simulink model "LgrstClsRStEnCtrl"  (R2018b)
settings: Solver=FixedStepDiscrete  StartTime=0.0  StopTime=10.0  FixedStep=0.01  RelTol=1e-3
undefined symbols (not defined in the file or in its folder): data, KeSMSw4SSecRwRtStLgrstOtwdInwdClosePos1_Val, KeSMSw4SSecRwRtStLgrstUpwdDnwdClosePos1_Val, KeSMSw4SSecRwRtStLgrstUpwdDnwdClosePos2_Val, SecRwRtStFtrstEn_Clear, SecRwRtStFtrstEn_Set, SecRwRtStLgrstInwdOtwdEn_Clear, SecRwRtStLgrstInwdOtwdEn_Set, SecRwRtStLgrstUpwdDnwdEn_Clear, SecRwRtStLgrstUpwdDnwdEn_Set
libraries: simulink x7
settings Model: Creator=sn2xws  LastModifiedBy=sn2xws
settings DataIOCC: SaveFormat=StructureWithTime
settings OptimizationCC: DefaultParameterBehavior=Inlined  EnhancedBackFolding=on  PassReuseOutputArgsAs=Individual arguments  ZeroExternalMemoryAtStartup=off  ZeroInternalMemoryAtStartup=off  OptimizeBlockOrder=speed  DifferentSizesBufferReuse=on  OptimizationCustomize=off
settings DebuggingCC: ParameterTunabilityLossMsg=error
settings ModelReferenceCC: ModelReferenceNumInstancesAllowed=Single
settings SFSimCC: MATLABDynamicMemAlloc=off
settings RTWCC: SystemTargetFile=autosar.tlc  GenCodeOnly=on  TemplateMakefile=ert_default_tmf  Description=AUTOSAR  GenerateReport=on  IncludeHyperlinkInReport=on  LaunchReport=on  GenerateTraceInfo=on  GenerateTraceReport=on  GenerateTraceReportSl=on  GenerateTraceReportSf=on  GenerateTraceReportEml=on
settings CodeAppCC: ForceParamTrailComments=on  IgnoreCustomStorageClasses=off  OperatorAnnotations=on  SimulinkDataObjDesc=on  SFDataObjDesc=on  InsertBlockDesc=on
settings STFCustomTargetCC: TargetLangStandard=C99 (ISO)  MultiwordLength=256  ParMdlRefBuildCompliant=on  CompOptLevelCompliant=on  IncludeMdlTerminateFcn=off  CombineOutputUpdateFcns=on  SuppressErrorStatus=on  ERTCustomFileBanners=on  SupportNonFinite=off  SupportComplex=off  SupportContinuousTime=off  SupportNonInlinedSFcns=off  RemoveResetFunc=on  MATLABClassNameForMDSCustomization=Simulink.SoftwareTarget.ERTCustomization  AutosarCompliant=on  UseToolchainInfoCompliant=on  LookupTableObjectStructAxisOrder=2,1,3,4,...  LUTObjectStructOrderEvenSpacing=Size,Table,Breakpoints  SystemTargetFile=autosar.tlc
settings ERTTargetCC: TargetLangStandard=C99 (ISO)  ConcurrentExecutionCompliant=off  IncludeMdlTerminateFcn=off  SuppressErrorStatus=on  SupportNonFinite=off  SupportComplex=off  ModelStepFunctionPrototypeControlCompliant=off  CPPClassGenCompliant=off  AutosarCompliant=on  LookupTableObjectStructAxisOrder=2,1,3,4,...  LUTObjectStructOrderEvenSpacing=Size,Table,Breakpoints  InlinedParameterPlacement=NonHierarchical  ERTCustomFileTemplate=example_file_process.tlc  ERTFilePackagingFormat=Compact

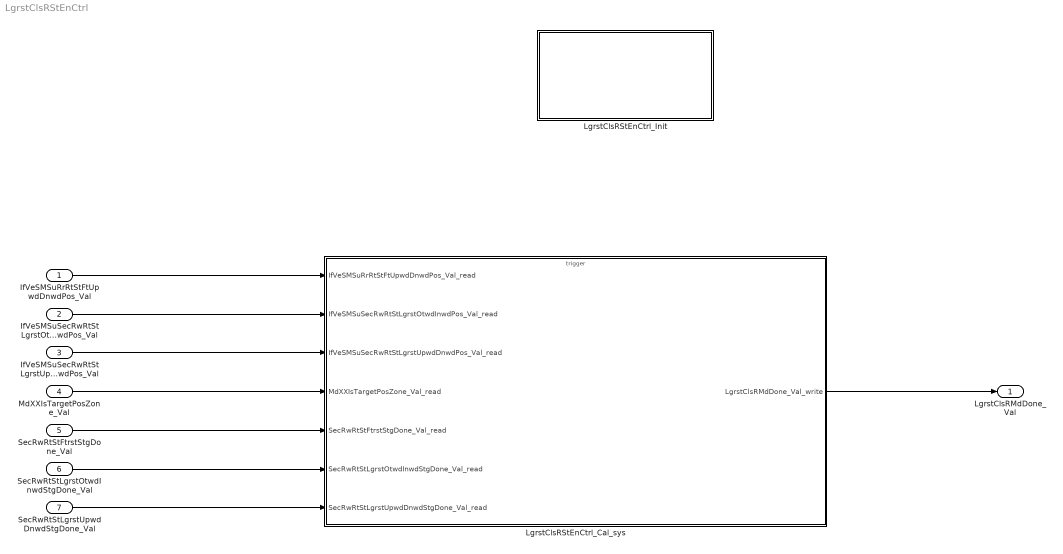
== system LgrstClsRStEnCtrl ==
  IfVeSMSuRrRtStFtUpwdDnwdPos_Val : Inport  OutDataTypeStr=uint16  PortDimensions=1
  IfVeSMSuSecRwRtStLgrstOtwdInwdPos_Val : Inport  Port=2  OutDataTypeStr=uint16  PortDimensions=1
  IfVeSMSuSecRwRtStLgrstUpwdDnwdPos_Val : Inport  Port=3  OutDataTypeStr=uint16  PortDimensions=1
  MdXXIsTargetPosZone_Val : Inport  Port=4  OutDataTypeStr=uint32  PortDimensions=1
  SecRwRtStFtrstStgDone_Val : Inport  Port=5  OutDataTypeStr=boolean  PortDimensions=1
  SecRwRtStLgrstOtwdInwdStgDone_Val : Inport  Port=6  OutDataTypeStr=boolean  PortDimensions=1
  SecRwRtStLgrstUpwdDnwdStgDone_Val : Inport  Port=7  OutDataTypeStr=boolean  PortDimensions=1
  LgrstClsRStEnCtrl_Cal_sys : Subsystem
  LgrstClsRStEnCtrl_Init : Subsystem
  LgrstClsRMdDone_Val : Outport  OutDataTypeStr=uint8  PortDimensions=1
  wires:
  IfVeSMSuRrRtStFtUpwdDnwdPos_Val/1 -> LgrstClsRStEnCtrl_Cal_sys/1(IfVeSMSuRrRtStFtUpwdDnwdPos_Val_read)
  IfVeSMSuSecRwRtStLgrstOtwdInwdPos_Val/1 -> LgrstClsRStEnCtrl_Cal_sys/2(IfVeSMSuSecRwRtStLgrstOtwdInwdPos_Val_read)
  IfVeSMSuSecRwRtStLgrstUpwdDnwdPos_Val/1 -> LgrstClsRStEnCtrl_Cal_sys/3(IfVeSMSuSecRwRtStLgrstUpwdDnwdPos_Val_read)
  MdXXIsTargetPosZone_Val/1 -> LgrstClsRStEnCtrl_Cal_sys/4(MdXXIsTargetPosZone_Val_read)
  SecRwRtStFtrstStgDone_Val/1 -> LgrstClsRStEnCtrl_Cal_sys/5(SecRwRtStFtrstStgDone_Val_read)
  SecRwRtStLgrstOtwdInwdStgDone_Val/1 -> LgrstClsRStEnCtrl_Cal_sys/6(SecRwRtStLgrstOtwdInwdStgDone_Val_read)
  SecRwRtStLgrstUpwdDnwdStgDone_Val/1 -> LgrstClsRStEnCtrl_Cal_sys/7(SecRwRtStLgrstUpwdDnwdStgDone_Val_read)
  LgrstClsRStEnCtrl_Cal_sys/1(LgrstClsRMdDone_Val_write) -> LgrstClsRMdDone_Val/1

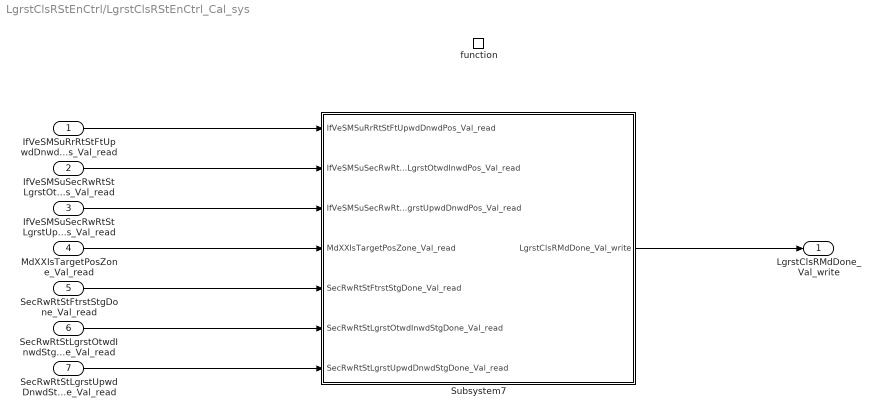
== system LgrstClsRStEnCtrl/LgrstClsRStEnCtrl_Cal_sys ==
  IfVeSMSuRrRtStFtUpwdDnwdPos_Val_read : Inport
  IfVeSMSuSecRwRtStLgrstOtwdInwdPos_Val_read : Inport  Port=2
  IfVeSMSuSecRwRtStLgrstUpwdDnwdPos_Val_read : Inport  Port=3
  MdXXIsTargetPosZone_Val_read : Inport  Port=4
  SecRwRtStFtrstStgDone_Val_read : Inport  Port=5
  SecRwRtStLgrstOtwdInwdStgDone_Val_read : Inport  Port=6
  SecRwRtStLgrstUpwdDnwdStgDone_Val_read : Inport  Port=7
  function : TriggerPort  TriggerType=function-call  IsSimulinkFunction=on  FunctionName=LgrstClsRStEnCtrl_Cal  VariantControl=(inherit)
  Subsystem7 : Subsystem
  LgrstClsRMdDone_Val_write : Outport
      settings: EnsureOutportIsVirtual=on
  wires:
  IfVeSMSuRrRtStFtUpwdDnwdPos_Val_read/1 -> Subsystem7/1(IfVeSMSuRrRtStFtUpwdDnwdPos_Val_read)
  IfVeSMSuSecRwRtStLgrstOtwdInwdPos_Val_read/1 -> Subsystem7/2(IfVeSMSuSecRwRtStLgrstOtwdInwdPos_Val_read)
  IfVeSMSuSecRwRtStLgrstUpwdDnwdPos_Val_read/1 -> Subsystem7/3(IfVeSMSuSecRwRtStLgrstUpwdDnwdPos_Val_read)
  MdXXIsTargetPosZone_Val_read/1 -> Subsystem7/4(MdXXIsTargetPosZone_Val_read)
  SecRwRtStFtrstStgDone_Val_read/1 -> Subsystem7/5(SecRwRtStFtrstStgDone_Val_read)
  SecRwRtStLgrstOtwdInwdStgDone_Val_read/1 -> Subsystem7/6(SecRwRtStLgrstOtwdInwdStgDone_Val_read)
  SecRwRtStLgrstUpwdDnwdStgDone_Val_read/1 -> Subsystem7/7(SecRwRtStLgrstUpwdDnwdStgDone_Val_read)
  Subsystem7/1(LgrstClsRMdDone_Val_write) -> LgrstClsRMdDone_Val_write/1

== system LgrstClsRStEnCtrl/LgrstClsRStEnCtrl_Init ==
  Event Listener : EventListener  EventName=reset

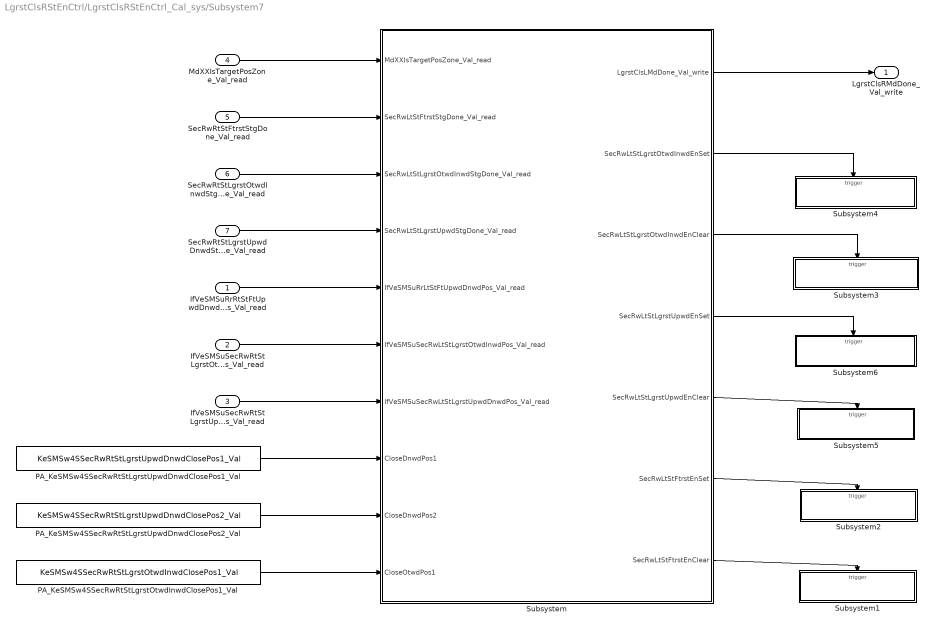
== system LgrstClsRStEnCtrl/LgrstClsRStEnCtrl_Cal_sys/Subsystem7 ==
  IfVeSMSuRrRtStFtUpwdDnwdPos_Val_read : Inport
  IfVeSMSuSecRwRtStLgrstOtwdInwdPos_Val_read : Inport  Port=2
  IfVeSMSuSecRwRtStLgrstUpwdDnwdPos_Val_read : Inport  Port=3
  MdXXIsTargetPosZone_Val_read : Inport  Port=4
  SecRwRtStFtrstStgDone_Val_read : Inport  Port=5
  SecRwRtStLgrstOtwdInwdStgDone_Val_read : Inport  Port=6
  SecRwRtStLgrstUpwdDnwdStgDone_Val_read : Inport  Port=7
  PA_KeSMSw4SSecRwRtStLgrstOtwdInwdClosePos1_Val : Constant  Value=KeSMSw4SSecRwRtStLgrstOtwdInwdClosePos1_Val
  PA_KeSMSw4SSecRwRtStLgrstUpwdDnwdClosePos1_Val : Constant  Value=KeSMSw4SSecRwRtStLgrstUpwdDnwdClosePos1_Val
  PA_KeSMSw4SSecRwRtStLgrstUpwdDnwdClosePos2_Val : Constant  Value=KeSMSw4SSecRwRtStLgrstUpwdDnwdClosePos2_Val
  Subsystem : Subsystem
  Subsystem1 : Subsystem
  Subsystem2 : Subsystem
  Subsystem3 : Subsystem
  Subsystem4 : Subsystem
  Subsystem5 : Subsystem
  Subsystem6 : Subsystem
  LgrstClsRMdDone_Val_write : Outport
      settings: EnsureOutportIsVirtual=on
  wires:
  SecRwRtStLgrstUpwdDnwdStgDone_Val_read/1 -> Subsystem/4(SecRwLtStLgrstUpwdStgDone_Val_read)
  SecRwRtStLgrstOtwdInwdStgDone_Val_read/1 -> Subsystem/3(SecRwLtStLgrstOtwdInwdStgDone_Val_read)
  IfVeSMSuSecRwRtStLgrstUpwdDnwdPos_Val_read/1 -> Subsystem/7(IfVeSMSuSecRwLtStLgrstUpwdDnwdPos_Val_read)
  MdXXIsTargetPosZone_Val_read/1 -> Subsystem/1(MdXXIsTargetPosZone_Val_read)
  Subsystem/1(LgrstClsLMdDone_Val_write) -> LgrstClsRMdDone_Val_write/1
  Subsystem/7(SecRwLtStFtrstEnClear) -> Subsystem1/Trigger
  SecRwRtStFtrstStgDone_Val_read/1 -> Subsystem/2(SecRwLtStFtrstStgDone_Val_read)
  Subsystem/4(SecRwLtStLgrstUpwdEnSet) -> Subsystem6/Trigger
  PA_KeSMSw4SSecRwRtStLgrstUpwdDnwdClosePos2_Val/1 -> Subsystem/9(CloseDnwdPos2)
  Subsystem/2(SecRwLtStLgrstOtwdInwdEnSet) -> Subsystem4/Trigger
  Subsystem/6(SecRwLtStFtrstEnSet) -> Subsystem2/Trigger
  IfVeSMSuRrRtStFtUpwdDnwdPos_Val_read/1 -> Subsystem/5(IfVeSMSuRrLtStFtUpwdDnwdPos_Val_read)
  Subsystem/3(SecRwLtStLgrstOtwdInwdEnClear) -> Subsystem3/Trigger
  IfVeSMSuSecRwRtStLgrstOtwdInwdPos_Val_read/1 -> Subsystem/6(IfVeSMSuSecRwLtStLgrstOtwdInwdPos_Val_read)
  PA_KeSMSw4SSecRwRtStLgrstOtwdInwdClosePos1_Val/1 -> Subsystem/10(CloseOtwdPos1)
  PA_KeSMSw4SSecRwRtStLgrstUpwdDnwdClosePos1_Val/1 -> Subsystem/8(CloseDnwdPos1)
  Subsystem/5(SecRwLtStLgrstUpwdEnClear) -> Subsystem5/Trigger

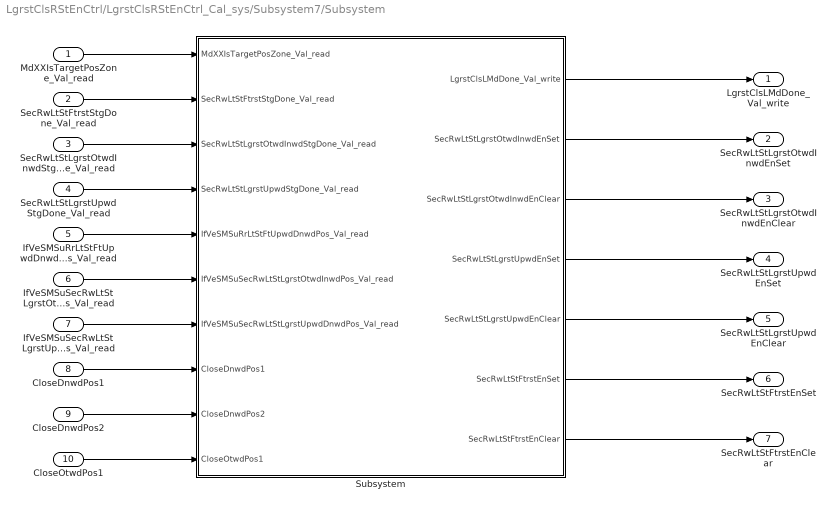
== system LgrstClsRStEnCtrl/LgrstClsRStEnCtrl_Cal_sys/Subsystem7/Subsystem ==
  MdXXIsTargetPosZone_Val_read : Inport
  SecRwLtStFtrstStgDone_Val_read : Inport  Port=2
  SecRwLtStLgrstOtwdInwdStgDone_Val_read : Inport  Port=3
  SecRwLtStLgrstUpwdStgDone_Val_read : Inport  Port=4
  IfVeSMSuRrLtStFtUpwdDnwdPos_Val_read : Inport  Port=5
  IfVeSMSuSecRwLtStLgrstOtwdInwdPos_Val_read : Inport  Port=6
  IfVeSMSuSecRwLtStLgrstUpwdDnwdPos_Val_read : Inport  Port=7
  CloseDnwdPos1 : Inport  Port=8
  CloseDnwdPos2 : Inport  Port=9
  CloseOtwdPos1 : Inport  Port=10
  Subsystem : Subsystem
  LgrstClsLMdDone_Val_write : Outport
      settings: EnsureOutportIsVirtual=on
  SecRwLtStLgrstOtwdInwdEnSet : Outport  Port=2
  SecRwLtStLgrstOtwdInwdEnClear : Outport  Port=3
  SecRwLtStLgrstUpwdEnSet : Outport  Port=4
  SecRwLtStLgrstUpwdEnClear : Outport  Port=5
  SecRwLtStFtrstEnSet : Outport  Port=6
  SecRwLtStFtrstEnClear : Outport  Port=7
  wires:
  MdXXIsTargetPosZone_Val_read/1 -> Subsystem/1(MdXXIsTargetPosZone_Val_read)
  SecRwLtStFtrstStgDone_Val_read/1 -> Subsystem/2(SecRwLtStFtrstStgDone_Val_read)
  SecRwLtStLgrstOtwdInwdStgDone_Val_read/1 -> Subsystem/3(SecRwLtStLgrstOtwdInwdStgDone_Val_read)
  SecRwLtStLgrstUpwdStgDone_Val_read/1 -> Subsystem/4(SecRwLtStLgrstUpwdStgDone_Val_read)
  Subsystem/1(LgrstClsLMdDone_Val_write) -> LgrstClsLMdDone_Val_write/1
  IfVeSMSuSecRwLtStLgrstOtwdInwdPos_Val_read/1 -> Subsystem/6(IfVeSMSuSecRwLtStLgrstOtwdInwdPos_Val_read)
  IfVeSMSuRrLtStFtUpwdDnwdPos_Val_read/1 -> Subsystem/5(IfVeSMSuRrLtStFtUpwdDnwdPos_Val_read)
  IfVeSMSuSecRwLtStLgrstUpwdDnwdPos_Val_read/1 -> Subsystem/7(IfVeSMSuSecRwLtStLgrstUpwdDnwdPos_Val_read)
  CloseDnwdPos1/1 -> Subsystem/8(CloseDnwdPos1)
  CloseDnwdPos2/1 -> Subsystem/9(CloseDnwdPos2)
  CloseOtwdPos1/1 -> Subsystem/10(CloseOtwdPos1)
  Subsystem/7(SecRwLtStFtrstEnClear) -> SecRwLtStFtrstEnClear/1
  Subsystem/3(SecRwLtStLgrstOtwdInwdEnClear) -> SecRwLtStLgrstOtwdInwdEnClear/1
  Subsystem/2(SecRwLtStLgrstOtwdInwdEnSet) -> SecRwLtStLgrstOtwdInwdEnSet/1
  Subsystem/6(SecRwLtStFtrstEnSet) -> SecRwLtStFtrstEnSet/1
  Subsystem/4(SecRwLtStLgrstUpwdEnSet) -> SecRwLtStLgrstUpwdEnSet/1
  Subsystem/5(SecRwLtStLgrstUpwdEnClear) -> SecRwLtStLgrstUpwdEnClear/1

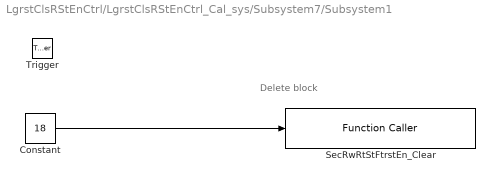
== system LgrstClsRStEnCtrl/LgrstClsRStEnCtrl_Cal_sys/Subsystem7/Subsystem1 ==
  note: Delete block
  Trigger : TriggerPort  TriggerType=function-call  VariantControl=Variant  PortDimensions=1
  Constant : Constant  Value=18  OutDataTypeStr=uint8
  SecRwRtStFtrstEn_Clear : FunctionCaller  FunctionPrototype=SecRwRtStFtrstEn_Clear(data)  InputArgumentSpecifications=uint8(1)
  wires:
  Constant/1 -> SecRwRtStFtrstEn_Clear/1

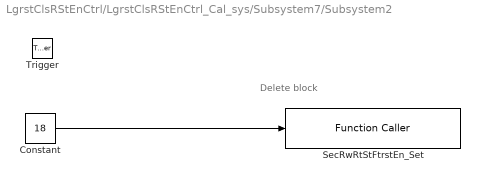
== system LgrstClsRStEnCtrl/LgrstClsRStEnCtrl_Cal_sys/Subsystem7/Subsystem2 ==
  note: Delete block
  Trigger : TriggerPort  TriggerType=function-call  VariantControl=Variant  PortDimensions=1
  Constant : Constant  Value=18  OutDataTypeStr=uint8
  SecRwRtStFtrstEn_Set : FunctionCaller  FunctionPrototype=SecRwRtStFtrstEn_Set(data)  InputArgumentSpecifications=uint8(1)
  wires:
  Constant/1 -> SecRwRtStFtrstEn_Set/1

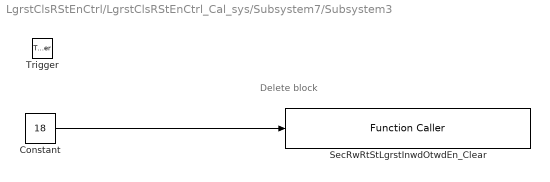
== system LgrstClsRStEnCtrl/LgrstClsRStEnCtrl_Cal_sys/Subsystem7/Subsystem3 ==
  note: Delete block
  Trigger : TriggerPort  TriggerType=function-call  VariantControl=Variant  PortDimensions=1
  Constant : Constant  Value=18  OutDataTypeStr=uint8
  SecRwRtStLgrstInwdOtwdEn_Clear : FunctionCaller  FunctionPrototype=SecRwRtStLgrstInwdOtwdEn_Clear(data)  InputArgumentSpecifications=uint8(1)
  wires:
  Constant/1 -> SecRwRtStLgrstInwdOtwdEn_Clear/1

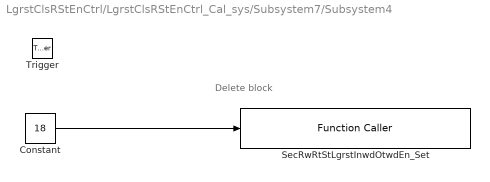
== system LgrstClsRStEnCtrl/LgrstClsRStEnCtrl_Cal_sys/Subsystem7/Subsystem4 ==
  note: Delete block
  Trigger : TriggerPort  TriggerType=function-call  VariantControl=Variant  PortDimensions=1
  Constant : Constant  Value=18  OutDataTypeStr=uint8
  SecRwRtStLgrstInwdOtwdEn_Set : FunctionCaller  FunctionPrototype=SecRwRtStLgrstInwdOtwdEn_Set(data)  InputArgumentSpecifications=uint8(1)
  wires:
  Constant/1 -> SecRwRtStLgrstInwdOtwdEn_Set/1

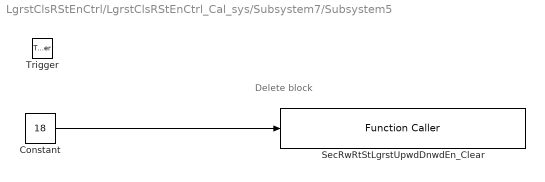
== system LgrstClsRStEnCtrl/LgrstClsRStEnCtrl_Cal_sys/Subsystem7/Subsystem5 ==
  note: Delete block
  Trigger : TriggerPort  TriggerType=function-call  VariantControl=Variant  PortDimensions=1
  Constant : Constant  Value=18  OutDataTypeStr=uint8
  SecRwRtStLgrstUpwdDnwdEn_Clear : FunctionCaller  FunctionPrototype=SecRwRtStLgrstUpwdDnwdEn_Clear(data)  InputArgumentSpecifications=uint8(1)
  wires:
  Constant/1 -> SecRwRtStLgrstUpwdDnwdEn_Clear/1

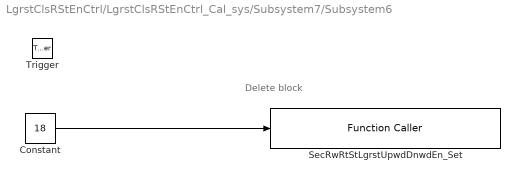
== system LgrstClsRStEnCtrl/LgrstClsRStEnCtrl_Cal_sys/Subsystem7/Subsystem6 ==
  note: Delete block
  Trigger : TriggerPort  TriggerType=function-call  VariantControl=Variant  PortDimensions=1
  Constant : Constant  Value=18  OutDataTypeStr=uint8
  SecRwRtStLgrstUpwdDnwdEn_Set : FunctionCaller  FunctionPrototype=SecRwRtStLgrstUpwdDnwdEn_Set(data)  InputArgumentSpecifications=uint8(1)
  wires:
  Constant/1 -> SecRwRtStLgrstUpwdDnwdEn_Set/1

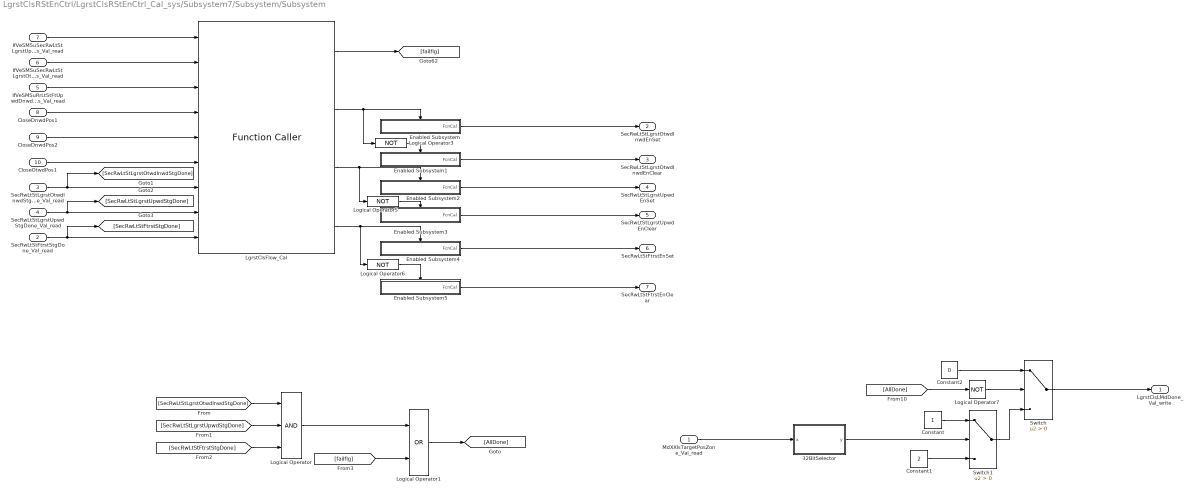
== system LgrstClsRStEnCtrl/LgrstClsRStEnCtrl_Cal_sys/Subsystem7/Subsystem/Subsystem ==
  MdXXIsTargetPosZone_Val_read : Inport
  SecRwLtStFtrstStgDone_Val_read : Inport  Port=2
  SecRwLtStLgrstOtwdInwdStgDone_Val_read : Inport  Port=3
  SecRwLtStLgrstUpwdStgDone_Val_read : Inport  Port=4
  IfVeSMSuRrLtStFtUpwdDnwdPos_Val_read : Inport  Port=5
  IfVeSMSuSecRwLtStLgrstOtwdInwdPos_Val_read : Inport  Port=6
  IfVeSMSuSecRwLtStLgrstUpwdDnwdPos_Val_read : Inport  Port=7
  CloseDnwdPos1 : Inport  Port=8
  CloseDnwdPos2 : Inport  Port=9
  CloseOtwdPos1 : Inport  Port=10
  32BitSelector : Subsystem  mask(32 Bit Selector){BitNum=18}
      mask prompts: BitNum "Select Bit Number"
      mask help: Allows selection of a particular bit (0-31) out of a packed word up to 32 bits long. Output will be true if the bit number selected via the mask parameter is equal to one.
      mask TypeOptions BitNum: 0 | 1 | 2 | 3 | 4 | 5 | 6 | 7 | 8 | 9 | 10 | 11 | 12 | 13 | 14 | 15 | 16 | 17 | 18 | 19 | 20 | 21 | 22 | 23 | 24 | 25 | 26 | 27 | 28 | 29 | 30 | 31
      mask Display:
      | text(0.5, 0.8,'BIT','horizontalAlignment','center')
      | text(0.5, 0.5,'SELECTOR','horizontalAlignment','center')
      | text(0.5, 0.2,['-- Bit ',char(get_param(gcb,'BitNum')),' --'],'horizontalAlignment','center')
  Constant : Constant  OutDataTypeStr=uint8
  Constant1 : Constant  Value=2  OutDataTypeStr=uint8
  Constant2 : Constant  Value=0  OutDataTypeStr=uint8
  Enabled Subsystem : Subsystem  TreatAsAtomicUnit=on
  Enabled Subsystem1 : Subsystem  TreatAsAtomicUnit=on
  Enabled Subsystem2 : Subsystem  TreatAsAtomicUnit=on
  Enabled Subsystem3 : Subsystem  TreatAsAtomicUnit=on
  Enabled Subsystem4 : Subsystem  TreatAsAtomicUnit=on
  Enabled Subsystem5 : Subsystem  TreatAsAtomicUnit=on
  LgrstClsFlow_Cal : FunctionCaller  FunctionPrototype=[Failflg,LgrstInwdOtwdEn,LgrstUpwdDnwdEn,FtrstEn] = LgrstClsFlow_Cal(LgrstUpwdDnwdPos,LgrstOtwdInwdPos,FtUpwdDnwdPos,CloseDnwdPos1,CloseDnwdPos2,CloseOtwdPos1,LgrstInwdStgDone,LgrstUpwdStgDone,FtrstStgDone)  InputArgumentSpecifications=uint16(1), uint16(1), uint16(1), uint16(1), uint16(1), uint16(1), boolean(true), boolean(true), boolean(true)  OutputArgumentSpecifications=boolean(true), boolean(true), boolean(true), boolean(true)
  Logical Operator : Logic  Inputs=3  AllPortsSameDT=off  OutDataTypeStr=boolean
  Logical Operator1 : Logic  Operator=OR  AllPortsSameDT=off  OutDataTypeStr=boolean
  Logical Operator{3,5..7} (4 alike) : Logic  Operator=NOT  AllPortsSameDT=off  OutDataTypeStr=boolean
  Switch : Switch  Criteria=u2 > Threshold
  Switch1 : Switch  Criteria=u2 > Threshold
  LgrstClsLMdDone_Val_write : Outport
      settings: EnsureOutportIsVirtual=on
  SecRwLtStLgrstOtwdInwdEnSet : Outport  Port=2
  SecRwLtStLgrstOtwdInwdEnClear : Outport  Port=3
  SecRwLtStLgrstUpwdEnSet : Outport  Port=4
  SecRwLtStLgrstUpwdEnClear : Outport  Port=5
  SecRwLtStFtrstEnSet : Outport  Port=6
  SecRwLtStFtrstEnClear : Outport  Port=7
  wires:
  SecRwLtStLgrstOtwdInwdStgDone_Val_read/1 -> [SecRwLtStLgrstOtwdInwdStgDone], LgrstClsFlow_Cal/7
  IfVeSMSuRrLtStFtUpwdDnwdPos_Val_read/1 -> LgrstClsFlow_Cal/3
  SecRwLtStFtrstStgDone_Val_read/1 -> LgrstClsFlow_Cal/9, [SecRwLtStFtrstStgDone]
  IfVeSMSuSecRwLtStLgrstUpwdDnwdPos_Val_read/1 -> LgrstClsFlow_Cal/1
  SecRwLtStLgrstUpwdStgDone_Val_read/1 -> LgrstClsFlow_Cal/8, [SecRwLtStLgrstUpwdStgDone]
  CloseDnwdPos1/1 -> LgrstClsFlow_Cal/4
  IfVeSMSuSecRwLtStLgrstOtwdInwdPos_Val_read/1 -> LgrstClsFlow_Cal/2
  LgrstClsFlow_Cal/1 -> [failflg]
  CloseOtwdPos1/1 -> LgrstClsFlow_Cal/6
  CloseDnwdPos2/1 -> LgrstClsFlow_Cal/5
  Enabled Subsystem/1(FcnCal) -> SecRwLtStLgrstOtwdInwdEnSet/1
  Enabled Subsystem1/1(FcnCal) -> SecRwLtStLgrstOtwdInwdEnClear/1
  Enabled Subsystem2/1(FcnCal) -> SecRwLtStLgrstUpwdEnSet/1
  Enabled Subsystem3/1(FcnCal) -> SecRwLtStLgrstUpwdEnClear/1
  Enabled Subsystem4/1(FcnCal) -> SecRwLtStFtrstEnSet/1
  Enabled Subsystem5/1(FcnCal) -> SecRwLtStFtrstEnClear/1
  [SecRwLtStLgrstOtwdInwdStgDone] -> Logical Operator/1
  [SecRwLtStLgrstUpwdStgDone] -> Logical Operator/2
  [SecRwLtStFtrstStgDone] -> Logical Operator/3
  [failflg] -> Logical Operator1/2
  Logical Operator/1 -> Logical Operator1/1
  [AllDone] -> Logical Operator7/1
  MdXXIsTargetPosZone_Val_read/1 -> 32BitSelector/1(x)
  Switch1/1 -> Switch/3
  Switch/1 -> LgrstClsLMdDone_Val_write/1
  Logical Operator1/1 -> [AllDone]
  Logical Operator3/1 -> Enabled Subsystem1/Enable
  Logical Operator6/1 -> Enabled Subsystem5/Enable
  LgrstClsFlow_Cal/3 -> Logical Operator5/1, Enabled Subsystem2/Enable
  Logical Operator5/1 -> Enabled Subsystem3/Enable
  LgrstClsFlow_Cal/4 -> Logical Operator6/1, Enabled Subsystem4/Enable
  LgrstClsFlow_Cal/2 -> Logical Operator3/1, Enabled Subsystem/Enable
  Constant2/1 -> Switch/1
  Constant/1 -> Switch1/1
  Constant1/1 -> Switch1/3
  Logical Operator7/1 -> Switch/2
  32BitSelector/1(y) -> Switch1/2

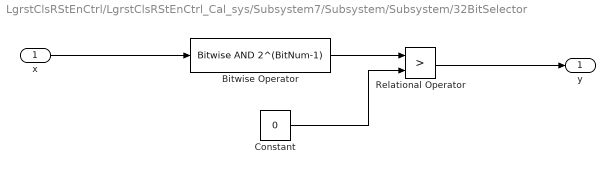
== system LgrstClsRStEnCtrl/LgrstClsRStEnCtrl_Cal_sys/Subsystem7/Subsystem/Subsystem/32BitSelector ==
  x : Inport
  Bitwise Operator : simulink/Logic and Bit Operations/Bitwise Operator  logicop=AND  UseBitMask=on  BitMask=2^(BitNum-1)  BitMaskRealWorld=Stored Integer
  Constant : Constant  Value=0  OutDataTypeStr=uint32
  Relational Operator : RelationalOperator  Operator=>  OutDataTypeStr=boolean  RndMeth=Simplest
  y : Outport
  wires:
  Relational Operator/1 -> y/1
  Constant/1 -> Relational Operator/2
  x/1 -> Bitwise Operator/1
  Bitwise Operator/1 -> Relational Operator/1

== system LgrstClsRStEnCtrl/LgrstClsRStEnCtrl_Cal_sys/Subsystem7/Subsystem/Subsystem/Enabled Subsystem ==
  Enable : EnablePort
  Function-Call Generator : simulink/Ports & Subsystems/Function-Call Generator  sample_time=-1  numberOfIterations=1
  FcnCal : Outport
  wires:
  Function-Call Generator/1 -> FcnCal/1

== system LgrstClsRStEnCtrl/LgrstClsRStEnCtrl_Cal_sys/Subsystem7/Subsystem/Subsystem/Enabled Subsystem1 ==
  Enable : EnablePort
  Function-Call Generator : simulink/Ports & Subsystems/Function-Call Generator  sample_time=-1  numberOfIterations=1
  FcnCal : Outport
  wires:
  Function-Call Generator/1 -> FcnCal/1

== system LgrstClsRStEnCtrl/LgrstClsRStEnCtrl_Cal_sys/Subsystem7/Subsystem/Subsystem/Enabled Subsystem2 ==
  Enable : EnablePort
  Function-Call Generator : simulink/Ports & Subsystems/Function-Call Generator  sample_time=-1  numberOfIterations=1
  FcnCal : Outport
  wires:
  Function-Call Generator/1 -> FcnCal/1

== system LgrstClsRStEnCtrl/LgrstClsRStEnCtrl_Cal_sys/Subsystem7/Subsystem/Subsystem/Enabled Subsystem3 ==
  Enable : EnablePort
  Function-Call Generator : simulink/Ports & Subsystems/Function-Call Generator  sample_time=-1  numberOfIterations=1
  FcnCal : Outport
  wires:
  Function-Call Generator/1 -> FcnCal/1

== system LgrstClsRStEnCtrl/LgrstClsRStEnCtrl_Cal_sys/Subsystem7/Subsystem/Subsystem/Enabled Subsystem4 ==
  Enable : EnablePort
  Function-Call Generator : simulink/Ports & Subsystems/Function-Call Generator  sample_time=-1  numberOfIterations=1
  FcnCal : Outport
  wires:
  Function-Call Generator/1 -> FcnCal/1

== system LgrstClsRStEnCtrl/LgrstClsRStEnCtrl_Cal_sys/Subsystem7/Subsystem/Subsystem/Enabled Subsystem5 ==
  Enable : EnablePort
  Function-Call Generator : simulink/Ports & Subsystems/Function-Call Generator  sample_time=-1  numberOfIterations=1
  FcnCal : Outport
  wires:
  Function-Call Generator/1 -> FcnCal/1
